simulink model "test_model_sw_hw"  (R2018a)
settings: Solver=FixedStepDiscrete  StartTime=0.0  StopTime=10.0  RelTol=1e-3
libraries: MoDesA_lib x1
settings Model: Creator=letras  LastModifiedBy=puya
settings OptimizationCC: DefaultParameterBehavior=Inlined  PassReuseOutputArgsAs=Individual arguments  ZeroInternalMemoryAtStartup=off
settings DebuggingCC: ParameterTunabilityLossMsg=error
settings HardwareCC: ProdBitPerPointer=32  ProdBitPerSizeT=32  ProdBitPerPtrDiffT=32  ProdLargestAtomicInteger=Long  ProdWordSize=32  ProdHWDeviceType=ARM Compatible->ARM 9
settings SFSimCC: MATLABDynamicMemAlloc=off
settings RTWCC: SystemTargetFile=ert.tlc  TemplateMakefile=ert_default_tmf  GenerateReport=on  IncludeHyperlinkInReport=on  LaunchReport=on  GenerateTraceInfo=on  GenerateTraceReport=on  GenerateTraceReportSl=on  GenerateTraceReportSf=on  GenerateTraceReportEml=on
settings CodeAppCC: ForceParamTrailComments=on  IgnoreCustomStorageClasses=off  OperatorAnnotations=on  SimulinkDataObjDesc=on  SFDataObjDesc=on  MATLABFcnDesc=on  InsertBlockDesc=on  StateflowObjectComments=on  MATLABSourceComments=on
settings ERTTargetCC: TargetLangStandard=C99 (ISO)  GenerateSampleERTMain=on  InlinedParameterPlacement=NonHierarchical  ERTCustomFileTemplate=example_file_process.tlc

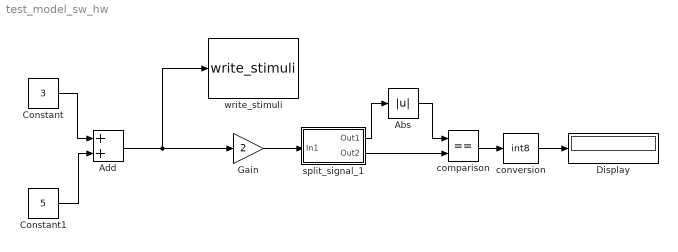
== system test_model_sw_hw ==
  Abs : Abs  Tag=hw_ip
  Add : Sum  Tag=sw
  Constant : Constant  Value=3
  Constant1 : Constant  Value=5
  Display : Display
  Gain : Gain  Tag=sw  Gain=2
  comparison : RelationalOperator  Tag=hw_ip  Operator===  OutDataTypeStr=boolean  RndMeth=Simplest
  conversion : DataTypeConversion  Tag=hw_ip  OutDataTypeStr=int8
  split_signal_1 : Subsystem  Tag=hw_ip
  write_stimuli : MoDesA_lib/write_stimuli  bound=1  instance=1
  wires:
  Constant1/1 -> Add/2
  Constant/1 -> Add/1
  split_signal_1/2(Out2) -> comparison/2
  comparison/1 -> conversion/1
  conversion/1 -> Display/1
  split_signal_1/1(Out1) -> Abs/1
  Abs/1 -> comparison/1
  Add/1 -> write_stimuli/1, Gain/1
  Gain/1 -> split_signal_1/1(In1)

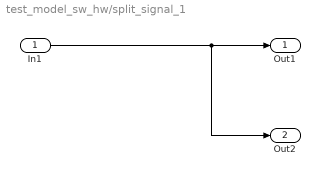
== system test_model_sw_hw/split_signal_1 ==
  In1 : Inport
  Out1 : Outport
  Out2 : Outport  Port=2
  wires:
  In1/1 -> Out2/1, Out1/1
